simulink model "FD_PITCH_COUPLED"  (R2019b)
settings: Solver=VariableStepAuto  StartTime=0.0  StopTime=10.0  RelTol=1e-3
undefined symbols (not defined in the file): Dm, Dt, g, Jp, k_pitch, k_yp, Mb
libraries: cstblocks x3
settings Model: Creator=lbend  LastModifiedBy=peter

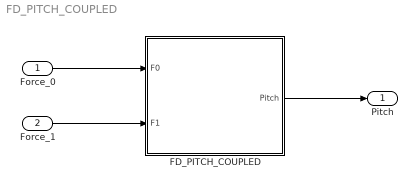
== system FD_PITCH_COUPLED ==
  Force_0 : Inport
  Force_1 : Inport  Port=2
  FD_PITCH_COUPLED : Subsystem
  Pitch : Outport
  wires:
  Force_0/1 -> FD_PITCH_COUPLED/1(F0)
  Force_1/1 -> FD_PITCH_COUPLED/2(F1)
  FD_PITCH_COUPLED/1(Pitch) -> Pitch/1

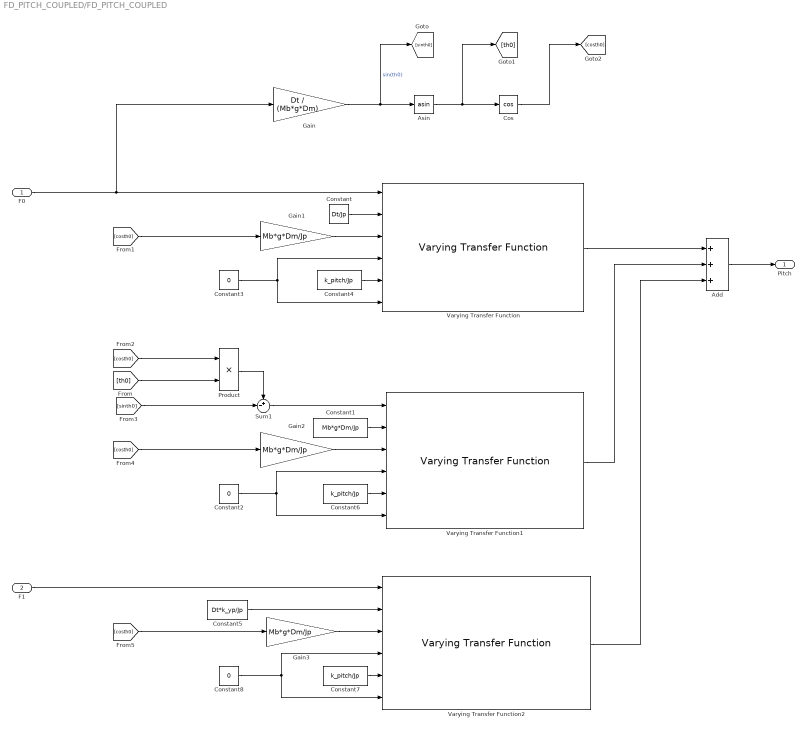
== system FD_PITCH_COUPLED/FD_PITCH_COUPLED ==
  F0 : Inport
  F1 : Inport  Port=2
  Add : Sum  Inputs=+++
  Asin : Trigonometry  Operator=asin
  Constant : Constant  Value=Dt/Jp  SampleTime=0
  Constant1 : Constant  Value=Mb*g*Dm/Jp  SampleTime=0
  Constant2 : Constant  Value=0  SampleTime=0
  Constant3 : Constant  Value=0  SampleTime=0
  Constant4 : Constant  Value=k_pitch/Jp  SampleTime=0
  Constant5 : Constant  Value=Dt*k_yp/Jp  SampleTime=0
  Constant6 : Constant  Value=k_pitch/Jp  SampleTime=0
  Constant7 : Constant  Value=k_pitch/Jp  SampleTime=0
  Constant8 : Constant  Value=0  SampleTime=0
  Cos : Trigonometry  Operator=cos
  Gain : Gain  Gain=Dt / (Mb*g*Dm)
  Gain1 : Gain  Gain=Mb*g*Dm/Jp
  Gain2 : Gain  Gain=Mb*g*Dm/Jp
  Gain3 : Gain  Gain=Mb*g*Dm/Jp
  Product : Product
  Sum1 : Sum  Inputs=+-|
  Varying Transfer Function : cstblocks/Linear Parameter Varying/Varying Transfer Function  N=2
      settings: SourceProductName=Control System Toolbox
  Varying Transfer Function1 : cstblocks/Linear Parameter Varying/Varying Transfer Function  N=2
      settings: SourceProductName=Control System Toolbox
  Varying Transfer Function2 : cstblocks/Linear Parameter Varying/Varying Transfer Function  N=2
      settings: SourceProductName=Control System Toolbox
  Pitch : Outport
  wires:
  Constant8/1 -> Varying Transfer Function2/4, Varying Transfer Function2/6
  Cos/1 -> [costh0]
  Constant3/1 -> Varying Transfer Function/4, Varying Transfer Function/6
  Gain2/1 -> Varying Transfer Function1/3
  Varying Transfer Function2/1 -> Add/3
  Asin/1 -> Cos/1, [th0]
  Constant7/1 -> Varying Transfer Function2/5
  Constant1/1 -> Varying Transfer Function1/2
  Constant2/1 -> Varying Transfer Function1/4, Varying Transfer Function1/6
  Constant6/1 -> Varying Transfer Function1/5
  Gain/1 -> [sinth0], Asin/1  "sin(th0)"
  [costh0] -> Gain1/1
  [th0] -> Product/2
  [costh0] -> Product/1
  Constant4/1 -> Varying Transfer Function/5
  F0/1 -> Varying Transfer Function/1, Gain/1
  [sinth0] -> Sum1/2
  Product/1 -> Sum1/1
  [costh0] -> Gain2/1
  Varying Transfer Function/1 -> Add/1
  Varying Transfer Function1/1 -> Add/2
  Gain1/1 -> Varying Transfer Function/3
  Sum1/1 -> Varying Transfer Function1/1
  Constant5/1 -> Varying Transfer Function2/2
  Constant/1 -> Varying Transfer Function/2
  [costh0] -> Gain3/1
  Add/1 -> Pitch/1
  Gain3/1 -> Varying Transfer Function2/3
  F1/1 -> Varying Transfer Function2/1
